simulink model "focusmodel"  (Simulink 7.9)
settings: Solver=ode45  StartTime=0.0  StopTime=10.0  RelTol=1e-6
undefined symbols (not defined in the file or in its folder): x, xdot
settings Model: Creator=abbas  LastModifiedBy=abbas
settings OptimizationCC: InlineInvariantSignals=on  InitFltsAndDblsToZero=on
settings DebuggingCC: SaveWithParameterizedLinksMsg=none  SignalResolutionControl=TryResolveAllWithWarning  SolverPrmCheckMsg=none  MultiTaskDSMMsg=warning  MultiTaskCondExecSysMsg=none  FcnCallInpInsideContextMsg=Use local settings  StrictBusMsg=None
settings RTWCC: IncludeERTFirstTime=on
settings GRTTargetCC: TargetFcnLib=ansi_tfl_tmw.mat  CombineOutputUpdateFcns=off  GRTInterface=on

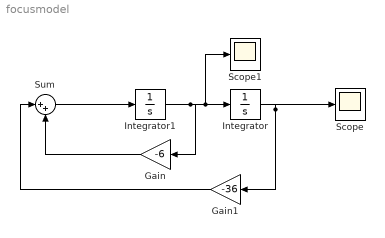
== system focusmodel ==
  Gain : Gain  Gain=-6
  Gain1 : Gain  Gain=-36
  Integrator : Integrator  InitialCondition=x
  Integrator1 : Integrator  InitialCondition=xdot
  Scope : Scope
      settings: SaveName=xfocus
  Scope1 : Scope
      settings: SaveName=xdotfocus
  Sum : Sum  Inputs=|++
  wires:
  Integrator1/1 -> Gain/1, Integrator/1, Scope1/1
  Integrator/1 -> Gain1/1, Scope/1
  Gain1/1 -> Sum/1
  Gain/1 -> Sum/2
  Sum/1 -> Integrator1/1
